simulink model "ESTS_FRIC_HILO_CONDLOG_test"  (R2024b)
settings: Solver=VariableStepAuto  StartTime=0.0  StopTime=10.0  RelTol=1e-3
libraries: ESTS_FRIC_HILO_CONDLOG x1
settings Model: Creator=blatak  LastModifiedBy=blatak

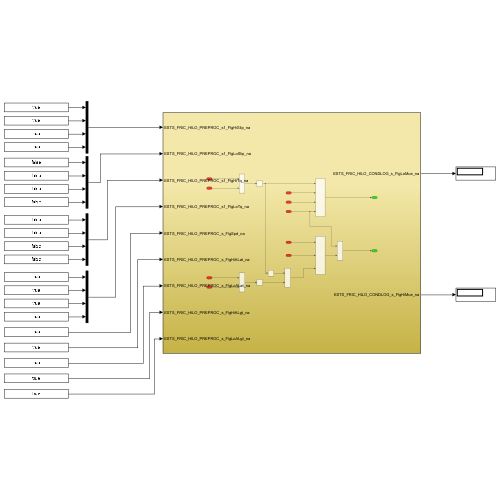
[thumbnail: Simulink's stored preview of the top-level diagram]
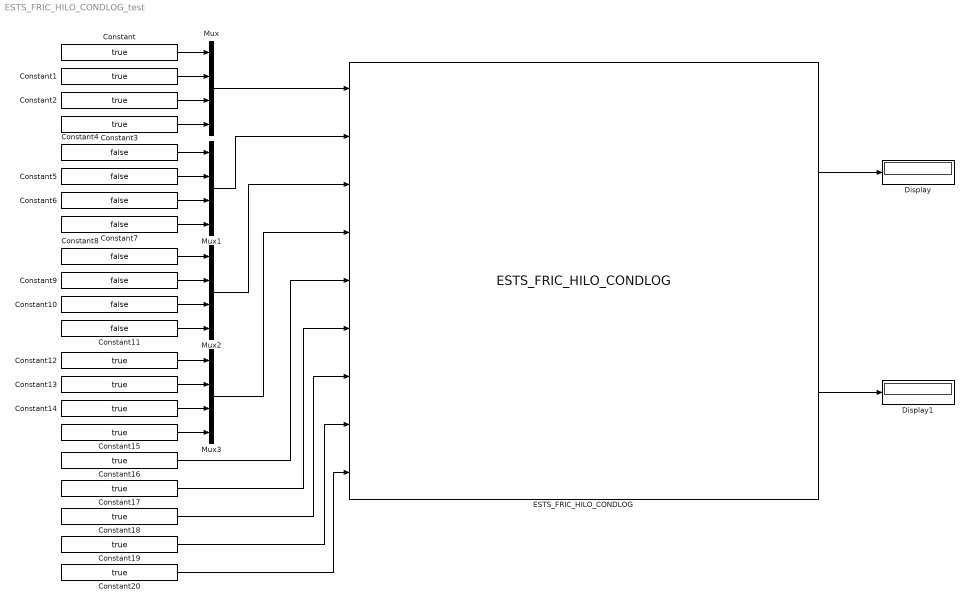
== system ESTS_FRIC_HILO_CONDLOG_test ==
  Constant{,1..3,12..20} (13 alike) : Constant  Value=true  OutDataTypeStr=boolean
  Constant{4..11} (8 alike) : Constant  Value=false  OutDataTypeStr=boolean
  Display : Display
  Display1 : Display
  ESTS_FRIC_HILO_CONDLOG : ESTS_FRIC_HILO_CONDLOG/ESTS_FRIC_HILO_CONDLOG/ESTS_FRIC_HILO_CONDLOG  SystemSampleTime=-1  VariantActivationTime=update diagram  AllowFlexibleInterface=on  Latency=0  AutoFrameSizeCalculation=off
  Mux{,1..3} (4 alike) : Mux
  wires:
  Mux/1 -> ESTS_FRIC_HILO_CONDLOG/1
  Constant/1 -> Mux/1
  Constant1/1 -> Mux/2
  Constant2/1 -> Mux/3
  Constant3/1 -> Mux/4
  Constant4/1 -> Mux1/1
  Constant5/1 -> Mux1/2
  Constant6/1 -> Mux1/3
  Constant7/1 -> Mux1/4
  Constant11/1 -> Mux2/4
  Constant10/1 -> Mux2/3
  Constant9/1 -> Mux2/2
  Constant8/1 -> Mux2/1
  Constant13/1 -> Mux3/2
  Constant15/1 -> Mux3/4
  Constant14/1 -> Mux3/3
  Constant12/1 -> Mux3/1
  Mux1/1 -> ESTS_FRIC_HILO_CONDLOG/2
  Mux2/1 -> ESTS_FRIC_HILO_CONDLOG/3
  Mux3/1 -> ESTS_FRIC_HILO_CONDLOG/4
  Constant20/1 -> ESTS_FRIC_HILO_CONDLOG/9
  Constant19/1 -> ESTS_FRIC_HILO_CONDLOG/8
  Constant18/1 -> ESTS_FRIC_HILO_CONDLOG/7
  Constant17/1 -> ESTS_FRIC_HILO_CONDLOG/6
  Constant16/1 -> ESTS_FRIC_HILO_CONDLOG/5
  ESTS_FRIC_HILO_CONDLOG/1 -> Display/1
  ESTS_FRIC_HILO_CONDLOG/2 -> Display1/1
